simulink model "System"  (R2021b)
settings: Solver=VariableStepAuto  StartTime=0.0  StopTime=10.0  RelTol=1e-3
model workspace (MAT data in the model file):
  x0 = Simulink.Parameter
  x0.Value = 0.3
  x0.DataType = 'auto'
  x0.Complexity = 'real'
  x0.Dimensions = [1 1]
settings Model: ParameterArgumentNames=x0  Creator=Hoorsana  LastModifiedBy=Hoorsana

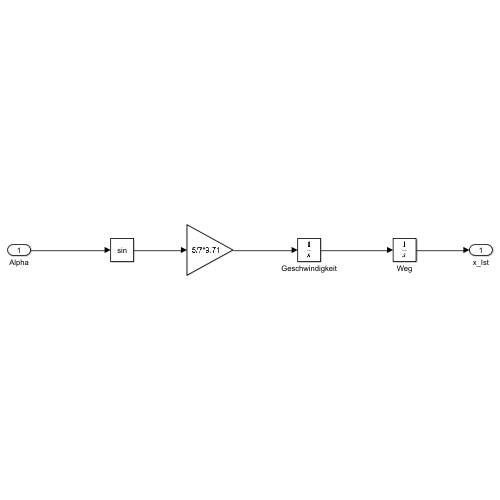
[thumbnail: Simulink's stored preview of the top-level diagram]
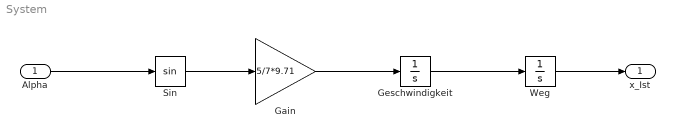
== system System ==
  Alpha : Inport
  Gain : Gain  Gain=5/7*9.71
  Geschwindigkeit : Integrator
  Sin : Trigonometry
  Weg : Integrator  InitialCondition=x0
  x_Ist : Outport  VectorParamsAs1DForOutWhenUnconnected=off
  wires:
  Geschwindigkeit/1 -> Weg/1
  Weg/1 -> x_Ist/1
  Sin/1 -> Gain/1
  Alpha/1 -> Sin/1
  Gain/1 -> Geschwindigkeit/1
